simulink model "tesla_model_s_async_R2019a"  (R2019a)
settings: Solver=ode23t  StartTime=0.0  StopTime=20  MaxStep=1/(60*100)  RelTol=1e-3
model workspace (MATLAB code in the model file):
  | L = 30e-3; % 30mH
  | R = 0.25; % Ohm armature resistance
  | tau_1 = L/R;
  | tau_source = 1/120;
  | tau1_div_tausource = tau_1/tau_source;
  | Vrms = 700;
  | Vd0 = 2/pi*sqrt(2)*Vrms
  | Vacpeak = Vrms*sqrt(2)
libraries: fl_lib x11, powerlib x9, nesl_utility x6, simulink x2, powerlib_meascontrol x1, eeSinGeneratorThreePhase x1
settings Model: EnablePacing=on  Creator=kjartan  LastModifiedBy=kjartan

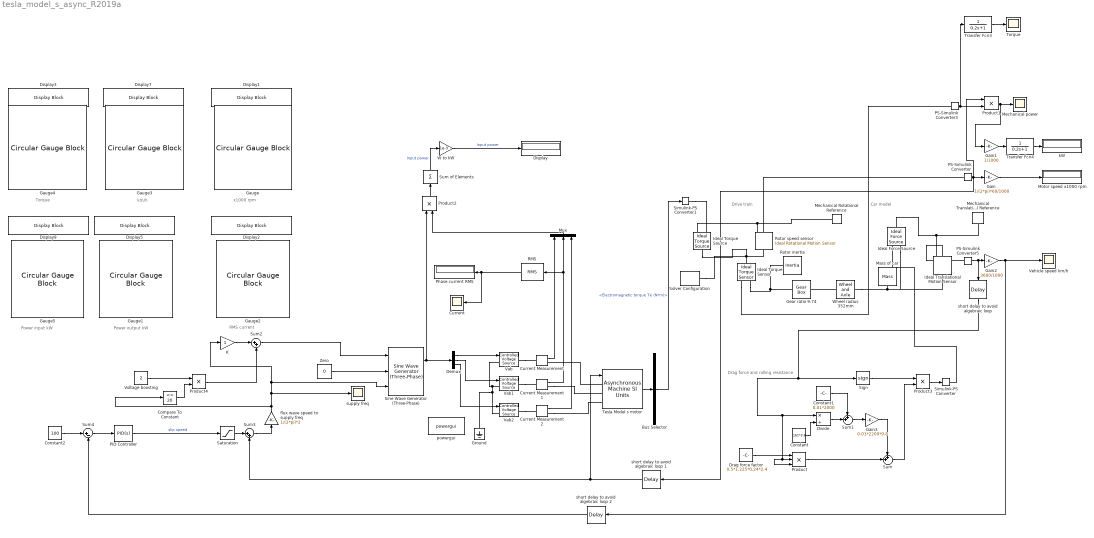
== system tesla_model_s_async_R2019a ==
  note: Car model
  note: Drive train
  note: x1000 rpm
  note: RMS current
  note: Power output kW
  note: Drag force and rolling resistance
  note: km/h
  note: Torque
  note: Power input kW
  Bus Selector : BusSelector  OutputSignals=Mechanical.Electromagnetic torque Te (N*m)
  Compare To Constant : simulink/Logic and Bit Operations/Compare To Constant  relop=<=  const=20  OutDataTypeStr=boolean
  Constant : Constant  Value=161*3.6
  Constant1 : Constant  Value=0.01*2000
  Constant2 : Constant  Value=100
  Current : Scope
  Current Measurement : powerlib/Measurements/Current Measurement  PhasorSimulation=off  OutputType=Complex  PSBequivalent=0
  Current Measurement1 : powerlib/Measurements/Current Measurement  PhasorSimulation=off  OutputType=Complex  PSBequivalent=0
  Current Measurement2 : powerlib/Measurements/Current Measurement  PhasorSimulation=off  OutputType=Complex  PSBequivalent=0
  Demux : Demux  Outputs=3
  Display : Display
  Display1 : DisplayBlock  LabelPosition=Hide  Format=short  Transparency=1  WebBlockId=340
  Display2 : DisplayBlock  LabelPosition=Hide  Format=short  Transparency=1  WebBlockId=352
  Display3 : DisplayBlock  LabelPosition=Hide  Format=short  Transparency=1  WebBlockId=472
  Display5 : DisplayBlock  LabelPosition=Hide  Format=short  Transparency=1  WebBlockId=364
  Display7 : DisplayBlock  LabelPosition=Hide  Format=short  Transparency=1  WebBlockId=414
  Display9 : DisplayBlock  LabelPosition=Hide  Format=short  Transparency=1  WebBlockId=526
  Divide : Product  Inputs=*/
  Drag force factor : Constant  Value=0.5*1.225*0.24*2.4
  Gain : Gain  Gain=1/(2*pi)*60/1000
  Gain1 : Gain  Gain=1/1000
  Gain2 : Gain  Gain=3600/1000
  Gain3 : Gain  Gain=0.01*2200*9.8
  Gauge : CircularGaugeBlock  ScaleMax=20  TickInterval=4  WebBlockId=118
  Gauge1 : CircularGaugeBlock  ScaleMax=600  TickInterval=100  WebBlockId=365
  Gauge2 : CircularGaugeBlock  ScaleMax=2000  TickInterval=200  WebBlockId=312
  Gauge3 : CircularGaugeBlock  ScaleMax=300  WebBlockId=415
  Gauge4 : CircularGaugeBlock  ScaleMax=800  TickInterval=100  WebBlockId=471
  Gauge5 : CircularGaugeBlock  ScaleMax=600  TickInterval=100  WebBlockId=525
  Gear ratio 9.74 : fl_lib/Mechanical/Mechanisms/Gear Box  ratio=9.744  t_in_specify=off  t_in_priority=None  t_in=0 N*m  t_in_nominal_specify=off  t_in_nominal_unit=N*m  t_in_nominal_value=1  t_out_specify=off  t_out_priority=None  t_out=0 N*m  t_out_nominal_specify=off  t_out_nominal_unit=N*m  t_out_nominal_value=1
  Ground : powerlib/Elements/Ground  LConnTagsString=a
  Ideal Force Source : fl_lib/Mechanical/Mechanical Sources/Ideal Force Source
  Ideal Torque Sensor : fl_lib/Mechanical/Mechanical Sensors/Ideal Torque Sensor
  Ideal Torque Source : fl_lib/Mechanical/Mechanical Sources/Ideal Torque Source
  Ideal Translational Motion Sensor : fl_lib/Mechanical/Mechanical Sensors/Ideal Translational Motion Sensor  offset=0 m
  K : Gain
  Mass of car : fl_lib/Mechanical/Translational Elements/Mass  mass=2200 kg  num_ports=foundation.enum.numPorts2.one  v_specify=off  v_priority=High  v=0 m/s  v_nominal_specify=off  v_nominal_unit=m/s  v_nominal_value=1  f_specify=off  f_priority=None  f=0 N  f_nominal_specify=off  f_nominal_unit=N  f_nominal_value=1
  Mechanical Rotational Reference : fl_lib/Mechanical/Rotational Elements/Mechanical Rotational Reference
  Mechanical Translational Reference : fl_lib/Mechanical/Translational Elements/Mechanical Translational Reference
  Mechanical power : Scope
  Motor speed x1000 rpm : Display
  Mux : Mux  Inputs=3
  PID Controller : simulink/Continuous/PID Controller  Controller=PID  Form=Parallel  TimeDomain=Continuous-time  SampleTime=-1  IntegratorMethod=Forward Euler  FilterMethod=Forward Euler  ControllerParametersSource=internal  P=0.3  I=0.01  D=0  UseFilter=on  N=100  TunerSelectOption=Transfer Function Based (PID Tuner App)  InitialConditionSource=internal  InitialConditionForIntegrator=0  InitialConditionForFilter=0  DifferentiatorICPrevScaledInput=0  ExternalReset=none  TrackingMode=off  Kt=1  LimitOutput=off  UpperSaturationLimit=inf  LowerSaturationLimit=-inf  LinearizeAsGain=on  AntiWindupMode=none  Kb=1  POutMin=[]  POutMax=[]  IOutMin=[]  IOutMax=[]  DOutMin=[]  DOutMax=[]  NOutMin=[]  NOutMax=[]  SumOutMin=[]  SumOutMax=[]  SaturationOutMin=[]  SaturationOutMax=[]  PParamMin=[]  PParamMax=[]  IParamMin=[]  IParamMax=[]  DParamMin=[]  DParamMax=[]  NParamMin=[]  NParamMax=[]  KbParamMin=[]  KbParamMax=[]  KtParamMin=[]  KtParamMax=[]  KbOutMin=[]  KbOutMax=[]  KtOutMin=[]  KtOutMax=[]  IntegratorOutMin=[]  IntegratorOutMax=[]  FilterOutMin=[]  FilterOutMax=[]  SumI1OutMin=[]  SumI1OutMax=[]  SumI2OutMin=[]  SumI2OutMax=[]  SumI3OutMin=[]  SumI3OutMax=[]  SumI4OutMin=[]  SumI4OutMax=[]  SumDOutMin=[]  SumDOutMax=[]  DifferentiatorOutMin=[]  DifferentiatorOutMax=[]  FilterDiffOutCoefMin=[]  FilterDiffOutCoefMax=[]  ReciprocalOutMin=[]  ReciprocalOutMax=[]  SumDenOutMin=[]  SumDenOutMax=[]  SumNumOutMin=[]  SumNumOutMax=[]  DivideOutMin=[]  DivideOutMax=[]  IntegratorContinuousStateAttributes=''  IntegratorStateMustResolveToSignalObject=off  IntegratorRTWStateStorageClass=Auto  FilterContinuousStateAttributes=''  FilterStateMustResolveToSignalObject=off  FilterRTWStateStorageClass=Auto  ParallelPVariant=InternalParameters  IdealPVariant=Disabled  IVariant=InternalParameters  DVariant=InternalParameters  IntegratorVariant=Continuous  SatVariant=Disabled  AWVariant=Passthrough  PCopyVariant=Disabled  TRVariant=Disabled  FdbkBlocksVariant=Forward  IdealPFdbkVariant=Disabled  SatFdbkVariant=Disabled  DerivativeFilterVariant=ContFilter  NVariant=InternalParameters  NCopyVariant=Disabled  FilterICVariant=InternalICsFilter  IntegratorICVariant=InternalICs  ExternalResetVariant=Disabled  TRSumVariant=Passthrough  SumFdbkVariant=Disabled  SumVariant=Sum_PID
  PS-Simulink Converter : nesl_utility/PS-Simulink Converter  PhysicalDomain=network_engine_domain  SubClassName=ps_output  LeftPortType=input  RightPortType=output  PseudoPeriodic=off  Frequencies=[]  Unit=inherit  AffineConversion=off
  PS-Simulink Converter3 : nesl_utility/PS-Simulink Converter  PhysicalDomain=network_engine_domain  SubClassName=ps_output  LeftPortType=input  RightPortType=output  PseudoPeriodic=off  Frequencies=[]  Unit=inherit  AffineConversion=off
  PS-Simulink Converter5 : nesl_utility/PS-Simulink Converter  PhysicalDomain=network_engine_domain  SubClassName=ps_output  LeftPortType=input  RightPortType=output  PseudoPeriodic=off  Frequencies=[]  Unit=inherit  AffineConversion=off
  Phase current RMS : Display
  Product : Product  Inputs=3
  Product{1..4} (4 alike) : Product
  RMS : powerlib_meascontrol/Measurements/RMS  TrueRMS=on  Freq=60  RMSInit=120  Ts=0
  Rotor inertia : fl_lib/Mechanical/Rotational Elements/Inertia  inertia=0.16 kg*m^2  num_ports=foundation.enum.numPorts2.one  w_specify=off  w_priority=High  w=0 rad/s  w_nominal_specify=off  w_nominal_unit=rad/s  w_nominal_value=1  t_specify=off  t_priority=None  t=0 N*m  t_nominal_specify=off  t_nominal_unit=N*m  t_nominal_value=1
  Rotor speed sensor : fl_lib/Mechanical/Mechanical Sensors/Ideal Rotational Motion Sensor  wrap_angle=simscape.enum.onoff.off  offset=0 rad
  Saturation : Saturate  UpperLimit=10  LowerLimit=0
  Sign : Signum
  Simulink-PS Converter : nesl_utility/Simulink-PS Converter  PhysicalDomain=network_engine_domain  SubClassName=ps_input  LeftPortType=input  RightPortType=output  PseudoPeriodic=off  Frequencies=[]  NoiseDistribution=none  NoiseParameters=[]  Unit=1  AffineConversion=off  FilteringAndDerivatives=provide  SimscapeFilterOrder=1  InputFilterTimeConstant=0.001  UdotUserProvided=0
  Simulink-PS Converter1 : nesl_utility/Simulink-PS Converter  PhysicalDomain=network_engine_domain  SubClassName=ps_input  LeftPortType=input  RightPortType=output  PseudoPeriodic=off  Frequencies=[]  NoiseDistribution=none  NoiseParameters=[]  Unit=1  AffineConversion=off  FilteringAndDerivatives=provide  SimscapeFilterOrder=1  InputFilterTimeConstant=0.001  UdotUserProvided=0
  Sine Wave Generator (Three-Phase) : eeSinGeneratorThreePhase/Sine Wave Generator (Three-Phase)  Ts=1/(40*280)
      settings: SourceProductBaseCode=PS
  Solver Configuration : nesl_utility/Solver Configuration  PhysicalDomain=network_engine_domain  SubClassName=solver  LeftPortType=input  RightPortType=generic  Tones=[]  Harmonics=[]  SimulateNoise=off  Profile=off  UseLocalSampling=off  EnableSwitchedLinearOptims=on  FrequencyDomain=off  UseCCode=off  RelTol=0.001  AbsTol=1e-06  MinStep=1e-09  ToWorkspace=off  RevertToSquareIcSolve=off  NumHomotopyIterations=100  PhasorMode=off  PhasorModeNumHarmonics=1  DoDC=off  ResidualTolerance=1e-09  UseLocalSolver=on  LocalSolverChoice=NE_BACKWARD_EULER_ADVANCER  LocalSolverSampleTime=1e-3  DoFixedCost=on  MaxNonlinIter=3  MaxModeIter=2  ComputeImpulses=off  ImpulseIterations=2  LinearAlgebra=auto  EquationFormulation=NE_TIME_EF  DelaysMemoryBudget=1024  AutomaticFiltering=on  FilteringTimeConstant=0.001  PartitionStorageMethod=AS_NEEDED  PartitionMemoryBudget=1024  PartitionMethod=ROBUST
  Sum : Sum  Inputs=++|
  Sum of Elements : Sum  Inputs=+
  Sum1 : Sum  Inputs=++|
  Sum2 : Sum  Inputs=|++
  Sum3 : Sum  Inputs=|++
  Sum4 : Sum  Inputs=|+-
  Tesla Model s motor : powerlib/Machines/Asynchronous Machine SI Units  RotorType=Squirrel-cage  PresetModel=No  MechanicalLoad=Speed w  ShowDetailedParameters=on  ReferenceFrame=Rotor  Units=SI  MeasurementBus=off  NominalParameters=[375, 230, 288]  Stator=[3e-3, 1.38e-6]  Rotor=[2e-3, 1.1052e-5]  Cage1=[0.4155 0.002066]  Cage2=[0.4168 0.0003495]  Lm=0.33157e-3  Mechanical=[0.05 0.005879 2]  PolePairs=2  InitialConditions=[0 0 0 0 0 0 0 0]  SimulateSaturation=off  Saturation=[14.03593122, 27.81365428, 53.79336849, 72.68890987, 97.98006896, 148.6815601, 215.7428561, 302.9841135, 428.7778367 ; 230, 322, 414, 460, 506, 552, 598, 644, 690]  LoadFlowParameters=1492000  TsPowergui=0  TsBlock=-1  IterativeModel=Trapezoidal non iterative  IterativeDiscreteModel=Trapezoidal non iterative  Pmec=1.492e+006
  Torque : Scope
  Transfer Fcn3 : TransferFcn  Denominator=[0.2 1]
  Transfer Fcn4 : TransferFcn  Denominator=[0.2 1]
  Vab : powerlib/Electrical Sources/Controlled Voltage Source  Description=source block  Initialize=on  Source_Type=AC  Amplitude=0  Phase=0  Frequency=0  Measurements=None
      settings: AttributesFormatString=\n
  Vab1 : powerlib/Electrical Sources/Controlled Voltage Source  Description=source block  Initialize=on  Source_Type=AC  Amplitude=0  Phase=0  Frequency=0  Measurements=None
      settings: AttributesFormatString=\n
  Vab2 : powerlib/Electrical Sources/Controlled Voltage Source  Description=source block  Initialize=on  Source_Type=AC  Amplitude=0  Phase=0  Frequency=0  Measurements=None
      settings: AttributesFormatString=\n
  Vehicle speed km/h : Scope
  Voltage boosting : Constant  Value=2
  W to kW : Gain  Gain=1e-3
  Wheel radius 352mm : fl_lib/Mechanical/Mechanisms/Wheel and Axle  R=0.352 m  or=1  t_specify=off  t_priority=None  t=0 N*m  t_nominal_specify=off  t_nominal_unit=N*m  t_nominal_value=1  f_specify=off  f_priority=None  f=0 N  f_nominal_specify=off  f_nominal_unit=N  f_nominal_value=1
  Zero : Constant  Value=0  OutDataTypeStr=Inherit: Inherit via back propagation
  flux wave speed to supply freq : Gain  Gain=1/(2*pi)*2
  kW : Display
  powergui : powerlib/powergui  Priority=1  SimulationMode=Continuous  SampleTime=50e-6  frequency=60  Iterations=50  frequencyindice=0  Pbase=100e6  ErrMax=1e-4  UnitsV=kV  UnitsW=MW  buscounter=0  FunctionMessages=off  echomessages=off  EnableUseOfTLC=off  CurrentSourceSwitches=off  DisableSnubberDevices=off  DisableRonSwitches=off  DisableVfSwitches=off  DisplayEquations=off  AutomaticDiscreteSolvers=off  SolverType=Tustin/Backward Euler (TBE)  Interpol=off  ExternalGateDelay=off  methode=off  Ts=100  x0status=blocks  SPID=on  SwTol=0  HookPort=off  NonlinearTolerance=1e-4  nMaxIteration=100  ContinueOnMaxIteration=off  RestoreLinks=warning  ResistiveCurrentMeasurement=off  Frange=[0:2:500]  Ylog=off  Xlog=on  ShowGrid=off  save=off  variable=ZData  structure=0  ZoomFFT=off  StartTime=0.0  cycles=1  DisplayStyle=1  fundamental=60  FreqAxis=off  MaxFrequency=1000  frequencyindicesteady=1  RmsSteady=1  display=off
  "short delay to avoid algebraic loop " : TransportDelay  DelayTime=1e-4
  short delay to avoid algebraic loop 1 : TransportDelay  DelayTime=1e-4
  short delay to avoid algebraic loop 2 : TransportDelay  DelayTime=1e-4
  supply freq : Scope
  wires:
  Gain/1 -> Motor speed x1000 rpm/1
  Product1/1 -> Gain1/1, Mechanical power/1
  "short delay to avoid algebraic loop "/1 -> Divide/1, Product/3, Product/2, Sign/1
  Drag force factor/1 -> Product/1
  Gain2/1 -> short delay to avoid algebraic loop 2/1, Vehicle speed km/h/1
  PS-Simulink Converter5/1 -> "short delay to avoid algebraic loop "/1, Gain2/1
  Product/1 -> Sum/2
  Constant/1 -> Divide/2
  Divide/1 -> Sum1/2
  Constant1/1 -> Sum1/1
  Sum1/1 -> Gain3/1
  Gain3/1 -> Sum/1
  Sign/1 -> Product3/1
  Sum/1 -> Product3/2
  Product3/1 -> Simulink-PS Converter/1
  Zero/1 -> Sine Wave Generator (Three-Phase)/2
  Sum2/1 -> Sine Wave Generator (Three-Phase)/1
  K/1 -> Sum2/1
  PS-Simulink Converter3/1 -> Transfer Fcn3/1, Product1/2
  Transfer Fcn3/1 -> Torque/1
  Gain1/1 -> Transfer Fcn4/1
  Transfer Fcn4/1 -> kW/1
  PID Controller/1 -> Saturation/1  "slip speed"
  Sum3/1 -> flux wave speed to supply freq/1
  flux wave speed to supply freq/1 -> K/1, Sine Wave Generator (Three-Phase)/3, supply freq/1, Compare To Constant/1
  Voltage boosting/1 -> Product4/1
  Product4/1 -> Sum2/2
  Compare To Constant/1 -> Product4/2
  short delay to avoid algebraic loop 1/1 -> Tesla Model s motor/1, Sum3/2
  Saturation/1 -> Sum3/1
  Constant2/1 -> Sum4/1
  Sum4/1 -> PID Controller/1
  short delay to avoid algebraic loop 2/1 -> Sum4/2
  Tesla Model s motor/1 -> Bus Selector/1
  Demux/1 -> Vab/1
  W to kW/1 -> Display/1  "Input power"
  Demux/2 -> Vab1/1
  Demux/3 -> Vab2/1
  Mux/1 -> Product2/2
  PS-Simulink Converter/1 -> short delay to avoid algebraic loop 1/1, Gain/1, Product1/1
  Product2/1 -> Sum of Elements/1
  Sine Wave Generator (Three-Phase)/1 -> Demux/1, Product2/1
  Current Measurement1/1 -> RMS/1, Mux/2
  Current Measurement2/1 -> Mux/3
  Current Measurement/1 -> Mux/1
  Bus Selector/1 -> Simulink-PS Converter1/1  "<Electromagnetic torque Te (N*m)>"
  RMS/1 -> Current/1, Phase current RMS/1
  Sum of Elements/1 -> W to kW/1  "Input power"
  connections:
  PS-Simulink Converter/LConn1 -- Rotor speed sensor/RConn2
  Ideal Torque Sensor/RConn2 -- PS-Simulink Converter3/LConn1
  Mechanical Rotational Reference/LConn1 -- Ideal Torque Source/RConn2 -- Rotor speed sensor/RConn1
  Rotor speed sensor/LConn1 -- Solver Configuration/RConn1 -- Ideal Torque Source/LConn1 -- Ideal Torque Sensor/LConn1
  Wheel radius 352mm/LConn1 -- Gear ratio 9.74/RConn1
  Wheel radius 352mm/RConn1 -- Ideal Force Source/RConn2 -- Ideal Translational Motion Sensor/LConn1 -- Mass of car/LConn1
  Ideal Torque Sensor/RConn1 -- Gear ratio 9.74/LConn1 -- Rotor inertia/LConn1
  Ideal Translational Motion Sensor/RConn1 -- Ideal Force Source/LConn1 -- Mechanical Translational Reference/LConn1
  Ideal Translational Motion Sensor/RConn2 -- PS-Simulink Converter5/LConn1
  Simulink-PS Converter/RConn1 -- Ideal Force Source/RConn1
  Vab1/LConn1 -- Ground/LConn1 -- Vab2/LConn1 -- Vab/LConn1
  Current Measurement1/RConn1 -- Tesla Model s motor/LConn2
  Vab1/RConn1 -- Current Measurement1/LConn1
  Vab/RConn1 -- Current Measurement/LConn1
  Vab2/RConn1 -- Current Measurement2/LConn1
  Tesla Model s motor/LConn1 -- Current Measurement/RConn1
  Current Measurement2/RConn1 -- Tesla Model s motor/LConn3
  Simulink-PS Converter1/RConn1 -- Ideal Torque Source/RConn1
